simulink model "DZ_AC_easyFOC"  (R2019b)
settings: Solver=VariableStepAuto  StartTime=0.0  StopTime=15  RelTol=1e-3
undefined symbols (not defined in the file): alfa_beta, beta, fr_n, j, J, k_comp, ki_f, ki_I, ki_m, kp_f, kp_I, kp_m, Lkm, Lks, load_yn, magnitude, n0, np, rad_to_rpm, ref_speed, Rr, Rs, sigbuilder_block, T_1_amp, T_amp, tau_f
libraries: simulink x2
settings Model: Creator=denni  LastModifiedBy=denniszanutto

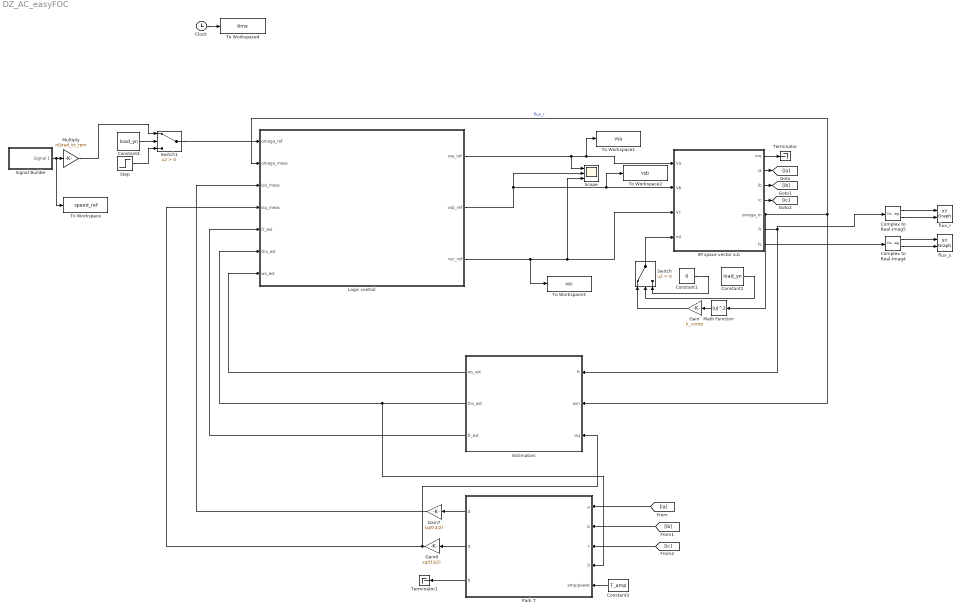
== system DZ_AC_easyFOC ==
  Clock : Clock
  Complex to Real-Imag4 : ComplexToRealImag
  Complex to Real-Imag5 : ComplexToRealImag
  Constant1 : Constant  Value=0
  Constant2 : Constant  Value=load_yn
  Constant3 : Constant  Value=T_amp
  Constant4 : Constant  Value=load_yn
  Estimators : Subsystem
  Gain : Gain  Gain=k_comp
  Gain7 : Gain  Gain=sqrt(3/2)
  Gain8 : Gain  Gain=sqrt(3/2)
  IM space vector a,b : Subsystem
  "Logic control " : Subsystem
  Math Function : Math  Operator=magnitude^2  SignedPower=off  SaturateOnIntegerOverflow=on
  Multiply : Gain  Gain=n0/rad_to_rpm
  Park T : Subsystem
  Scope : Scope  NumInputPorts=3
  Signal Builder : Subsystem  Tag=STV Subsys  LoadFcn=sigbuilder_block('load');  StartFcn=sigbuilder_block('start');  StopFcn=sigbuilder_block('stop');  ClipboardFcn=sigbuilder_block('clipboard');  mask(Sigbuilder block){tuvar=[0:10]}
      mask help: Simulink:masks:SigbuilderBlock_MD
      mask init:
      | if ~strcmp(get_param(bdroot(gcbh),'SimulationStatus'),'stopped') tuvar = sigbuilder_block('maskInit'); end
      settings: CopyFcn=sigbuilder_block('copy');  DeleteFcn=sigbuilder_block('delete');  ModelCloseFcn=sigbuilder_block('modelClose');  PreSaveFcn=sigbuilder_block('preSave');  PauseFcn=sigbuilder_block('pause');  ContinueFcn=sigbuilder_block('continue');  NameChangeFcn=sigbuilder_block('namechange');  OpenFcn=sigbuilder_block('open',[437.6 199.2 550.4 400 ]);  CloseFcn=sigbuilder_block('close');
      mask Display: plot(0, 0, 100, 100,[2, 2, 32, 32, 2], [68, 8, 8, 68, 68],[32, 2], [38, 38], [32, 19, 2],[53, 60, 44], [32, 17, 17, 2],[16, 16, 31, 31]);txt = getActiveGroup(gcbh);text(2, 100, txt,'verticalAlignment', 'top');
  Step : Step  Time=5*tau_f  After=ref_speed  SampleTime=0
  Switch : Switch  Criteria=u2 > Threshold
  Switch1 : Switch  Criteria=u2 > Threshold
  Terminator : Terminator
  Terminator1 : Terminator
  To Workspace : ToWorkspace  VariableName=speed_ref  SaveFormat=Timeseries  SampleTime=-1
  To Workspace1 : ToWorkspace  VariableName=vsa  SaveFormat=Timeseries  SampleTime=-1
  To Workspace2 : ToWorkspace  VariableName=vsb  SaveFormat=Timeseries  SampleTime=-1
  To Workspace3 : ToWorkspace  VariableName=vsc  SaveFormat=Timeseries  SampleTime=-1
  To Workspace4 : ToWorkspace  VariableName=time  SaveFormat=Timeseries  SampleTime=-1
  flux_r : simulink/Sinks/XY Graph  xmin=-4  xmax=4  ymin=-4  ymax=4  st=-1
  flux_s : simulink/Sinks/XY Graph  xmin=-5  xmax=5  ymin=-5  ymax=5  st=-1
  wires:
  "Logic control "/3(vsc_ref) -> To Workspace3/1, Scope/3, IM space vector a,b/3(Vc)
  "Logic control "/1(vsa_ref) -> Scope/1, To Workspace1/1, IM space vector a,b/1(Va)
  "Logic control "/2("vsb_ref ") -> Scope/2, To Workspace2/1, IM space vector a,b/2(Vb)
  IM space vector a,b/6(fr) -> Complex to Real-Imag5/1, Estimators/1(fr)
  Estimators/3("fr_est ") -> "Logic control "/5(fr_est)
  Math Function/1 -> Gain/1
  Estimators/1("ws_est ") -> "Logic control "/7(ws_est)
  Gain/1 -> Switch/1
  Switch/1 -> IM space vector a,b/4(ml)
  Constant1/1 -> Switch/3
  Constant2/1 -> Switch/2
  Complex to Real-Imag4/2 -> flux_s/2
  Complex to Real-Imag4/1 -> flux_s/1
  IM space vector a,b/7(fs) -> Complex to Real-Imag4/1
  Complex to Real-Imag5/2 -> flux_r/2
  Complex to Real-Imag5/1 -> flux_r/1
  IM space vector a,b/5("omega_m ") -> "Logic control "/2(omega_meas), Estimators/2("wm "), Math Function/1  "flux_r"
  IM space vector a,b/1("me ") -> Terminator/1
  IM space vector a,b/2(ia) -> [ia]
  IM space vector a,b/3(ib) -> [ib]
  IM space vector a,b/4(ic) -> [ic]
  Clock/1 -> To Workspace4/1
  Park T/3(0) -> Terminator1/1
  Estimators/2("ths_est ") -> Park T/4(fi), "Logic control "/6(ths_est)
  Constant3/1 -> Park T/5("amp/power ")
  Park T/1(d) -> Gain7/1
  Park T/2("q ") -> Gain8/1
  [ic] -> Park T/3("c ")
  [ib] -> Park T/2(b)
  [ia] -> Park T/1(a)
  Gain7/1 -> "Logic control "/3(isd_meas)
  Gain8/1 -> Estimators/3("isq "), "Logic control "/4(isq_meas)
  Constant4/1 -> Switch1/2
  Step/1 -> Switch1/3
  Switch1/1 -> "Logic control "/1(omega_ref)
  Signal Builder/1(Signal 1) -> To Workspace/1, Multiply/1
  Multiply/1 -> Switch1/1

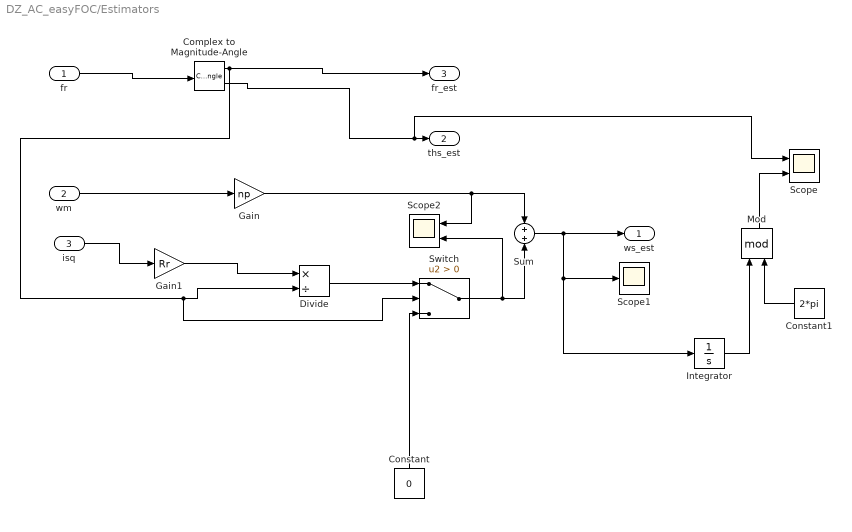
== system DZ_AC_easyFOC/Estimators ==
  fr : Inport
  "wm " : Inport  Port=2
  "isq " : Inport  Port=3
  Complex to Magnitude-Angle : ComplexToMagnitudeAngle
  Constant : Constant  Value=0
  Constant1 : Constant  Value=2*pi
  Divide : Product  Inputs=*/
  Gain : Gain  Gain=np
  Gain1 : Gain  Gain=Rr
  Integrator : Integrator
  Mod : Math  Operator=mod  SignedPower=off  SaturateOnIntegerOverflow=on
  Scope : Scope  NumInputPorts=2
  Scope1 : Scope
  Scope2 : Scope  NumInputPorts=2
  Sum : Sum
  Switch : Switch  Criteria=u2 > Threshold
  "ws_est " : Outport
  "ths_est " : Outport  Port=2
  "fr_est " : Outport  Port=3
  wires:
  fr/1 -> Complex to Magnitude-Angle/1
  Complex to Magnitude-Angle/2 -> Scope/1, "ths_est "/1
  "wm "/1 -> Gain/1
  Gain1/1 -> Divide/1
  "isq "/1 -> Gain1/1
  Complex to Magnitude-Angle/1 -> Switch/2, Divide/2, "fr_est "/1
  Divide/1 -> Switch/1
  Constant/1 -> Switch/3
  Switch/1 -> Scope2/2, Sum/2
  Gain/1 -> Scope2/1, Sum/1
  Sum/1 -> "ws_est "/1, Scope1/1, Integrator/1
  Constant1/1 -> Mod/2
  Integrator/1 -> Mod/1
  Mod/1 -> Scope/2

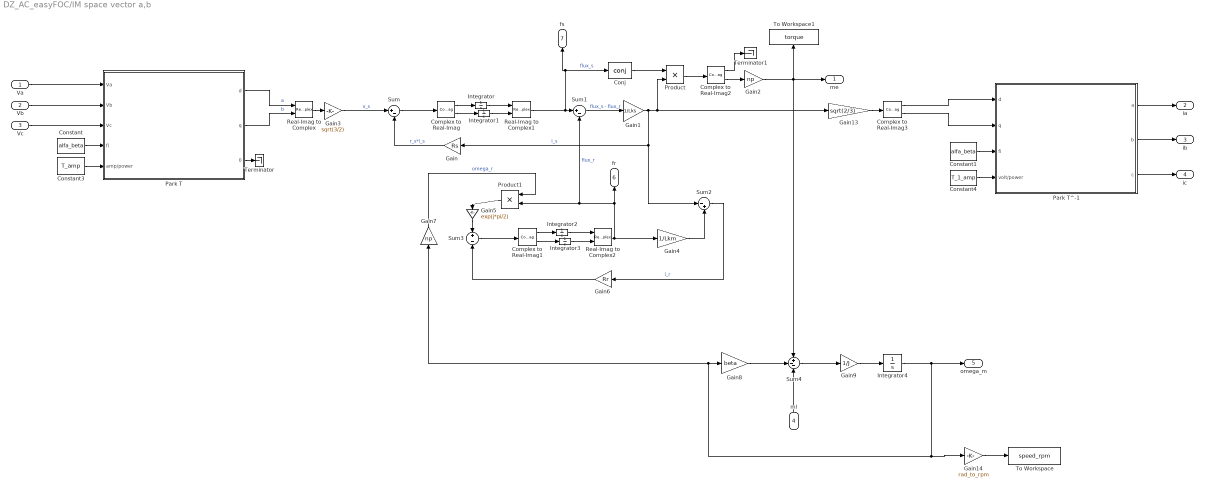
== system DZ_AC_easyFOC/IM space vector a,b ==
  Va : Inport
  Vb : Inport  Port=2
  Vc : Inport  Port=3
  ml : Inport  Port=4
  Complex to Real-Imag{,1..3} (4 alike) : ComplexToRealImag
  Conj : Math  Operator=conj  SignedPower=off  SaturateOnIntegerOverflow=on
  Constant : Constant  Value=alfa_beta
  Constant1 : Constant  Value=alfa_beta
  Constant3 : Constant  Value=T_amp
  Constant4 : Constant  Value=T_1_amp
  Gain : Gain  Gain=Rs
  Gain1 : Gain  Gain=1/Lks
  Gain13 : Gain  Gain=sqrt(2/3)
  Gain14 : Gain  Gain=rad_to_rpm
  Gain2 : Gain  Gain=np
  Gain3 : Gain  Gain=sqrt(3/2)
  Gain4 : Gain  Gain=1/Lkm
  Gain5 : Gain  Gain=exp(j*pi/2)
  Gain6 : Gain  Gain=Rr
  Gain7 : Gain  Gain=np
  Gain8 : Gain  Gain=beta
  Gain9 : Gain  Gain=1/J
  Integrator{,1..4} (5 alike) : Integrator
  Park T : Subsystem
  Park T^-1 : Subsystem
  Product : Product
  Product1 : Product
  Real-Imag to Complex : RealImagToComplex
  Real-Imag to Complex1 : RealImagToComplex
  Real-Imag to Complex2 : RealImagToComplex
  Sum : Sum  Inputs=|+-
  Sum1 : Sum  Inputs=|+-
  Sum2 : Sum  Inputs=|-+
  Sum3 : Sum  Inputs=+-
  Sum4 : Sum  Inputs=+--
  Terminator : Terminator
  Terminator1 : Terminator
  To Workspace : ToWorkspace  VariableName=speed_rpm  SaveFormat=Timeseries  SampleTime=-1
  To Workspace1 : ToWorkspace  VariableName=torque  SaveFormat=Timeseries  SampleTime=-1
  "me " : Outport
  ia : Outport  Port=2
  ib : Outport  Port=3
  ic : Outport  Port=4
  "omega_m " : Outport  Port=5
  fr : Outport  Port=6
  fs : Outport  Port=7
  wires:
  Vc/1 -> Park T/3("Vc ")
  Constant/1 -> Park T/4(fi)
  Constant3/1 -> Park T/5("amp/power ")
  Park T/1(d) -> Real-Imag to Complex/1  "a"
  Park T/2("q ") -> Real-Imag to Complex/2  "b"
  Real-Imag to Complex/1 -> Gain3/1
  Sum/1 -> Complex to Real-Imag/1
  Complex to Real-Imag/1 -> Integrator/1
  Complex to Real-Imag/2 -> Integrator1/1
  Integrator/1 -> Real-Imag to Complex1/1
  Integrator1/1 -> Real-Imag to Complex1/2
  Gain/1 -> Sum/2  "r_s*i_s"
  Real-Imag to Complex1/1 -> fs/1, Conj/1, Sum1/1  "flux_s"
  Sum1/1 -> Gain1/1  "flux_s - flux_r"
  Gain1/1 -> Product/2, Gain13/1, Sum2/1, Gain/1  "i_s"
  Conj/1 -> Product/1
  Complex to Real-Imag1/1 -> Integrator2/1
  Complex to Real-Imag1/2 -> Integrator3/1
  Integrator2/1 -> Real-Imag to Complex2/1
  Integrator3/1 -> Real-Imag to Complex2/2
  Gain4/1 -> Sum2/2
  Real-Imag to Complex2/1 -> fr/1, Sum1/2, Product1/2, Gain4/1  "flux_r"
  Sum3/1 -> Complex to Real-Imag1/1
  Gain5/1 -> Sum3/1
  Product1/1 -> Gain5/1
  Gain6/1 -> Sum3/2
  Sum2/1 -> Gain6/1  "i_r"
  ml/1 -> Sum4/3
  Sum4/1 -> Gain9/1
  Gain9/1 -> Integrator4/1
  Product/1 -> Complex to Real-Imag2/1
  Integrator4/1 -> "omega_m "/1, Gain14/1, Gain7/1, Gain8/1
  Gain2/1 -> "me "/1, To Workspace1/1, Sum4/1
  Va/1 -> Park T/1(Va)
  Vb/1 -> Park T/2(Vb)
  Gain8/1 -> Sum4/2
  Complex to Real-Imag2/2 -> Gain2/1
  Gain3/1 -> Sum/1  "v_s"
  Gain7/1 -> Product1/1  "omega_r"
  Gain13/1 -> Complex to Real-Imag3/1
  Complex to Real-Imag3/2 -> Park T^-1/2(q)
  Complex to Real-Imag3/1 -> Park T^-1/1(d)
  Constant1/1 -> Park T^-1/3(fi)
  Constant4/1 -> Park T^-1/4(volt/power)
  Park T^-1/1("a ") -> ia/1
  Park T^-1/2("b ") -> ib/1
  Park T^-1/3(c) -> ic/1
  Park T/3(0) -> Terminator/1
  Complex to Real-Imag2/1 -> Terminator1/1
  Gain14/1 -> To Workspace/1

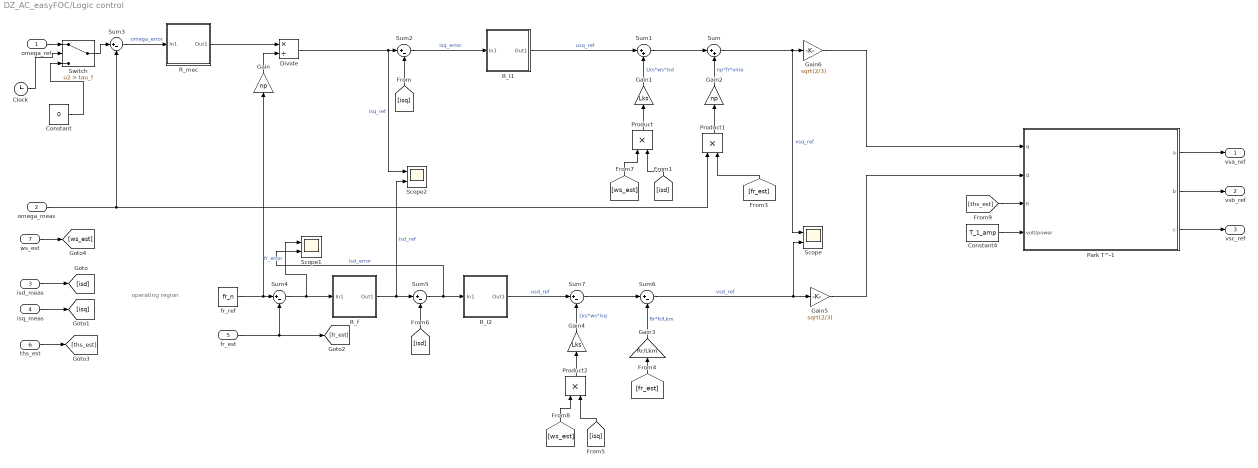
== system DZ_AC_easyFOC/Logic control  ==
  note: operating region
  omega_ref : Inport
  omega_meas : Inport  Port=2
  isd_meas : Inport  Port=3
  isq_meas : Inport  Port=4
  fr_est : Inport  Port=5
  ths_est : Inport  Port=6
  ws_est : Inport  Port=7
  Clock : Clock
  Constant : Constant  Value=0
  Constant4 : Constant  Value=T_1_amp
  Divide : Product  Inputs=*/
  Gain : Gain  Gain=np
  Gain1 : Gain  Gain=Lks
  Gain2 : Gain  Gain=np
  Gain3 : Gain  Gain=Rr/Lkm
  Gain4 : Gain  Gain=Lks
  Gain5 : Gain  Gain=sqrt(2/3)
  Gain6 : Gain  Gain=sqrt(2/3)
  Park T^-1 : Subsystem
  Product : Product
  Product1 : Product
  Product2 : Product
  R_I1 : Subsystem
  R_I2 : Subsystem
  "R_f " : Subsystem
  R_mec : Subsystem
  Scope : Scope  NumInputPorts=2
  Scope1 : Scope  NumInputPorts=2
  Scope2 : Scope  NumInputPorts=2
  Sum : Sum  Inputs=|++
  Sum1 : Sum  Inputs=|++
  Sum{2..7} (6 alike) : Sum  Inputs=|+-
  Switch : Switch  Criteria=u2 > Threshold  Threshold=tau_f
  "fr_ref " : Constant  Value=fr_n
  vsa_ref : Outport
  "vsb_ref " : Outport  Port=2
  vsc_ref : Outport  Port=3
  wires:
  Constant4/1 -> Park T^-1/4(volt/power)
  [ths_est] -> Park T^-1/3(fi)
  Sum/1 -> Scope/1, Gain6/1  "vsq_ref"
  Park T^-1/3(c) -> vsc_ref/1
  Sum1/1 -> Sum/1
  Sum3/1 -> R_mec/1(In1)  "omega_error"
  Gain/1 -> Divide/2
  ths_est/1 -> [ths_est]
  [isq] -> Sum2/2
  Product/1 -> Gain1/1
  [isd] -> Product/2
  omega_meas/1 -> Product1/1, Sum3/2
  Product1/1 -> Gain2/1
  "fr_ref "/1 -> Gain/1, Sum4/1
  fr_est/1 -> [fr_est], Sum4/2
  [fr_est] -> Product1/2
  Sum4/1 -> Scope1/1, "R_f "/1(In1)  "fr_error"
  "R_f "/1(Out1) -> Scope2/2, Sum5/1  "isd_ref"
  Sum5/1 -> Scope1/2, R_I2/1(In1)  "isd_error"
  Sum7/1 -> Sum6/1
  R_I2/1(Out1) -> Sum7/1  "usd_ref"
  Sum6/1 -> Scope/2, Gain5/1  "vsd_ref"
  [fr_est] -> Gain3/1
  Park T^-1/1("a ") -> vsa_ref/1
  Park T^-1/2("b ") -> "vsb_ref "/1
  [isq] -> Product2/2
  Product2/1 -> Gain4/1
  [isd] -> Sum5/2
  ws_est/1 -> [ws_est]
  [ws_est] -> Product/1
  [ws_est] -> Product2/1
  R_I1/1(Out1) -> Sum1/1  "usq_ref"
  Sum2/1 -> R_I1/1(In1)  "isq_error"
  R_mec/1(Out1) -> Divide/1
  Gain1/1 -> Sum1/2  "Lks*ws*isd"
  Gain2/1 -> Sum/2  "np*fr*ome"
  Gain4/1 -> Sum7/2  "Lks*ws*isq"
  Gain3/1 -> Sum6/2  "Rr*fr/Lkm"
  Divide/1 -> Scope2/1, Sum2/1  "isq_ref"
  Gain5/1 -> Park T^-1/2(d)
  Gain6/1 -> Park T^-1/1(q)
  isd_meas/1 -> [isd]
  isq_meas/1 -> [isq]
  omega_ref/1 -> Switch/1
  Switch/1 -> Sum3/1
  Constant/1 -> Switch/3
  Clock/1 -> Switch/2

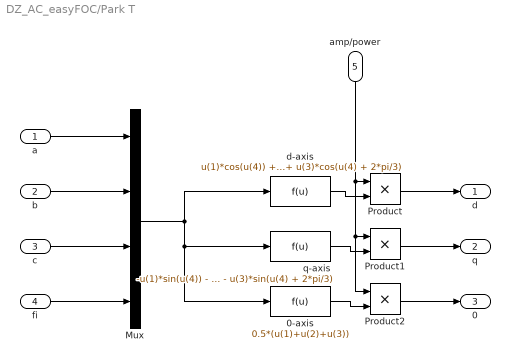
== system DZ_AC_easyFOC/Park T ==
  a : Inport
  b : Inport  Port=2
  "c " : Inport  Port=3
  fi : Inport  Port=4
  "amp/power " : Inport  Port=5
  0-axis : Fcn  Expr=0.5*(u(1)+u(2)+u(3))
  Mux : Mux
  Product : Product
  Product1 : Product
  Product2 : Product
  "d-axis " : Fcn  Expr=u(1)*cos(u(4)) + u(2)*cos(u(4) -2*pi/3) + u(3)*cos(u(4) + 2*pi/3)
  q-axis : Fcn  Expr=-u(1)*sin(u(4)) - u(2)*sin(u(4) -2*pi/3) - u(3)*sin(u(4) + 2*pi/3)
  d : Outport
  "q " : Outport  Port=2
  0 : Outport  Port=3
  wires:
  fi/1 -> Mux/4
  a/1 -> Mux/1
  b/1 -> Mux/2
  "c "/1 -> Mux/3
  Mux/1 -> "d-axis "/1, q-axis/1, 0-axis/1
  Product/1 -> d/1
  "d-axis "/1 -> Product/2
  Product1/1 -> "q "/1
  q-axis/1 -> Product1/2
  0-axis/1 -> Product2/2
  Product2/1 -> 0/1
  "amp/power "/1 -> Product2/1, Product1/1, Product/1

== system DZ_AC_easyFOC/Signal Builder ==
  Demux : Demux  Tag=STV Demux  Outputs=1
  FromWs : FromWorkspace  Tag=STV FromWs  VariableName=tuvar  SampleTime=0
      SigBuilderData=|
      | common.afterFinalStr = 'Extrapolate'
      | common.sampleTime = 0
      | dataSet.timeRange = [0 70]
      | dataSet.name = 'Group 1'
      | sbobj.Groups.Name = 'Group 1'
      | sbobj.Groups.Signals.Name = 'Signal 1'
      | sbobj.Groups.Signals.XData = [0 20 30 40 70]
      | sbobj.Groups.Signals.YData = [0 0.1 0.1 0.2 0.2]
      | sbobj.Groups.TimeRange = [0 70]
  Signal 1 : Outport  Tag=STV Outport
  wires:
  Demux/1 -> Signal 1/1
  FromWs/1 -> Demux/1

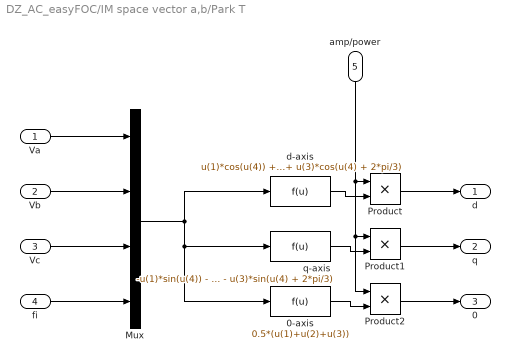
== system DZ_AC_easyFOC/IM space vector a,b/Park T ==
  Va : Inport
  Vb : Inport  Port=2
  "Vc " : Inport  Port=3
  fi : Inport  Port=4
  "amp/power " : Inport  Port=5
  0-axis : Fcn  Expr=0.5*(u(1)+u(2)+u(3))
  Mux : Mux
  Product : Product
  Product1 : Product
  Product2 : Product
  "d-axis " : Fcn  Expr=u(1)*cos(u(4)) + u(2)*cos(u(4) -2*pi/3) + u(3)*cos(u(4) + 2*pi/3)
  q-axis : Fcn  Expr=-u(1)*sin(u(4)) - u(2)*sin(u(4) -2*pi/3) - u(3)*sin(u(4) + 2*pi/3)
  d : Outport
  "q " : Outport  Port=2
  0 : Outport  Port=3
  wires:
  fi/1 -> Mux/4
  Va/1 -> Mux/1
  Vb/1 -> Mux/2
  "Vc "/1 -> Mux/3
  Mux/1 -> "d-axis "/1, q-axis/1, 0-axis/1
  Product/1 -> d/1
  "d-axis "/1 -> Product/2
  Product1/1 -> "q "/1
  q-axis/1 -> Product1/2
  0-axis/1 -> Product2/2
  Product2/1 -> 0/1
  "amp/power "/1 -> Product2/1, Product1/1, Product/1

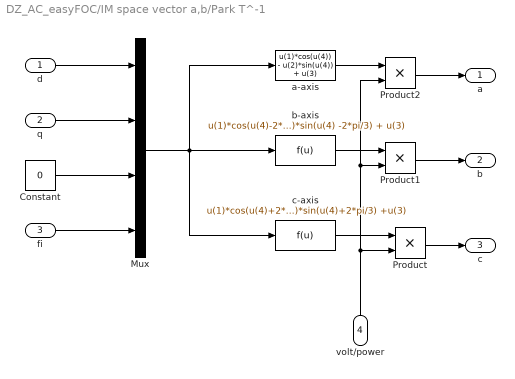
== system DZ_AC_easyFOC/IM space vector a,b/Park T^-1 ==
  d : Inport
  q : Inport  Port=2
  fi : Inport  Port=3
  volt/power : Inport  Port=4
  Constant : Constant  Value=0
  Mux : Mux
  Product : Product
  Product1 : Product
  Product2 : Product
  "a-axis " : Fcn  Expr=u(1)*cos(u(4)) - u(2)*sin(u(4)) + u(3)
  b-axis : Fcn  Expr=u(1)*cos(u(4)-2*pi/3) - u(2)*sin(u(4) -2*pi/3) + u(3)
  c-axis : Fcn  Expr=u(1)*cos(u(4)+2*pi/3) -u(2)*sin(u(4)+2*pi/3) +u(3)
  "a " : Outport
  "b " : Outport  Port=2
  c : Outport  Port=3
  wires:
  fi/1 -> Mux/4
  d/1 -> Mux/1
  q/1 -> Mux/2
  Mux/1 -> c-axis/1, b-axis/1, "a-axis "/1
  Constant/1 -> Mux/3
  volt/power/1 -> Product2/2, Product1/2, Product/2
  c-axis/1 -> Product/1
  Product/1 -> c/1
  Product1/1 -> "b "/1
  b-axis/1 -> Product1/1
  Product2/1 -> "a "/1
  "a-axis "/1 -> Product2/1

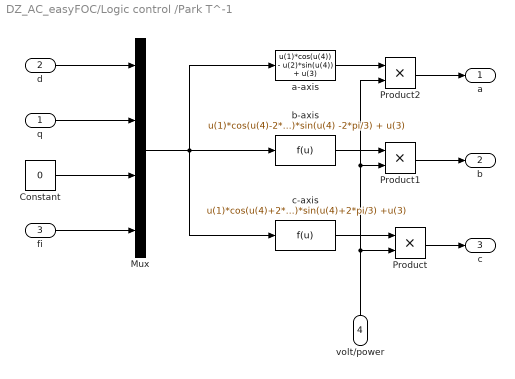
== system DZ_AC_easyFOC/Logic control /Park T^-1 ==
  q : Inport
  d : Inport  Port=2
  fi : Inport  Port=3
  volt/power : Inport  Port=4
  Constant : Constant  Value=0
  Mux : Mux
  Product : Product
  Product1 : Product
  Product2 : Product
  "a-axis " : Fcn  Expr=u(1)*cos(u(4)) - u(2)*sin(u(4)) + u(3)
  b-axis : Fcn  Expr=u(1)*cos(u(4)-2*pi/3) - u(2)*sin(u(4) -2*pi/3) + u(3)
  c-axis : Fcn  Expr=u(1)*cos(u(4)+2*pi/3) -u(2)*sin(u(4)+2*pi/3) +u(3)
  "a " : Outport
  "b " : Outport  Port=2
  c : Outport  Port=3
  wires:
  fi/1 -> Mux/4
  d/1 -> Mux/1
  q/1 -> Mux/2
  Mux/1 -> c-axis/1, b-axis/1, "a-axis "/1
  Constant/1 -> Mux/3
  volt/power/1 -> Product2/2, Product1/2, Product/2
  c-axis/1 -> Product/1
  Product/1 -> c/1
  Product1/1 -> "b "/1
  b-axis/1 -> Product1/1
  Product2/1 -> "a "/1
  "a-axis "/1 -> Product2/1

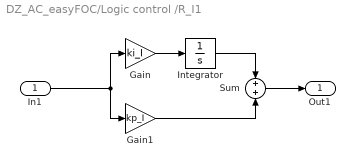
== system DZ_AC_easyFOC/Logic control /R_I1 ==
  In1 : Inport
  Gain : Gain  Gain=ki_I
  Gain1 : Gain  Gain=kp_I
  Integrator : Integrator
  Sum : Sum
  Out1 : Outport
  wires:
  Gain/1 -> Integrator/1
  In1/1 -> Gain/1, Gain1/1
  Integrator/1 -> Sum/1
  Gain1/1 -> Sum/2
  Sum/1 -> Out1/1

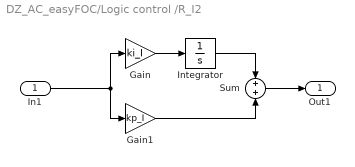
== system DZ_AC_easyFOC/Logic control /R_I2 ==
  In1 : Inport
  Gain : Gain  Gain=ki_I
  Gain1 : Gain  Gain=kp_I
  Integrator : Integrator
  Sum : Sum
  Out1 : Outport
  wires:
  Gain/1 -> Integrator/1
  In1/1 -> Gain/1, Gain1/1
  Integrator/1 -> Sum/1
  Gain1/1 -> Sum/2
  Sum/1 -> Out1/1

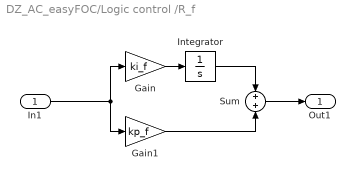
== system DZ_AC_easyFOC/Logic control /R_f  ==
  In1 : Inport
  Gain : Gain  Gain=ki_f
  Gain1 : Gain  Gain=kp_f
  Integrator : Integrator
  Sum : Sum
  Out1 : Outport
  wires:
  In1/1 -> Gain/1, Gain1/1
  Sum/1 -> Out1/1
  Gain/1 -> Integrator/1
  Integrator/1 -> Sum/1
  Gain1/1 -> Sum/2

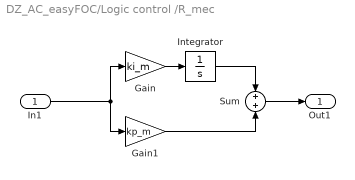
== system DZ_AC_easyFOC/Logic control /R_mec ==
  In1 : Inport
  Gain : Gain  Gain=ki_m
  Gain1 : Gain  Gain=kp_m
  Integrator : Integrator
  Sum : Sum
  Out1 : Outport
  wires:
  In1/1 -> Gain/1, Gain1/1
  Sum/1 -> Out1/1
  Gain/1 -> Integrator/1
  Integrator/1 -> Sum/1
  Gain1/1 -> Sum/2
